simulink model "min_ord"  (R2025a)
settings: Solver=VariableStepAuto  StartTime=0.0  StopTime=50  RelTol=1e-3
values from neighbouring files (symbols this model uses):
  A_hat = Abb- Ke_obs*Aab    [Controls_proj.m]
  A_real = double(A_real)    [Controls_proj.m]
  B_hat = A_hat*Ke_obs + Aba - Ke_obs*Aaa    [Controls_proj.m]
  B_real = double(B_real)    [Controls_proj.m]
  C_hat = zeros(6, 4)    [Controls_proj.m]
  C_sens = [1 0 0 0 0 0 ; 0 0 1 0 0 0]    [Controls_proj.m]
  D_hat = zeros(6, 2)    [Controls_proj.m]
  F_hat = Bb -Ke_obs*Ba    [Controls_proj.m]
  K = lqr(A_real,B_real,Q,R_lqr)    [Controls_proj.m]
libraries: simulink x2
settings Model: Creator=retqrd  LastModifiedBy=retqrd

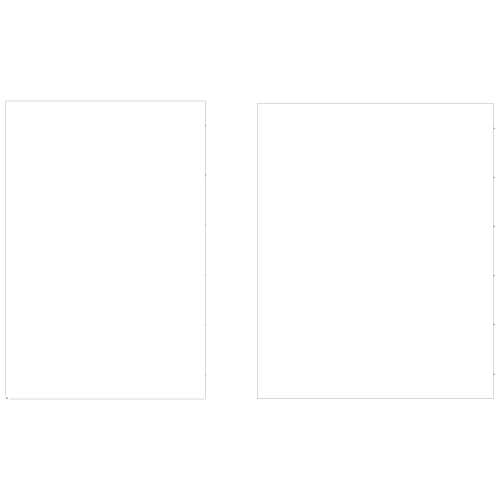
[thumbnail: Simulink's stored preview of the top-level diagram]
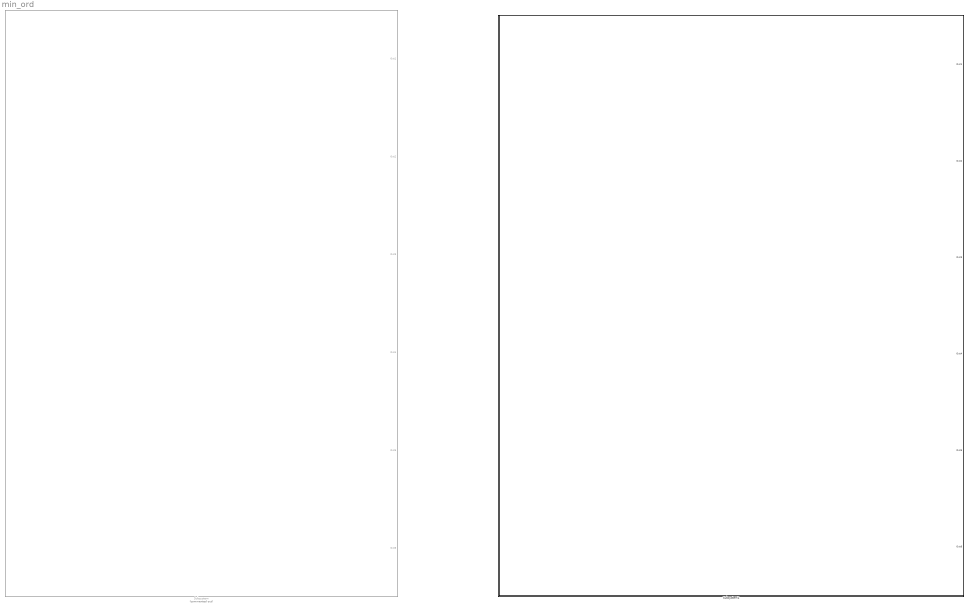
== system min_ord ==
  Subsystem : Subsystem  Commented=on
  Subsystem1 : Subsystem

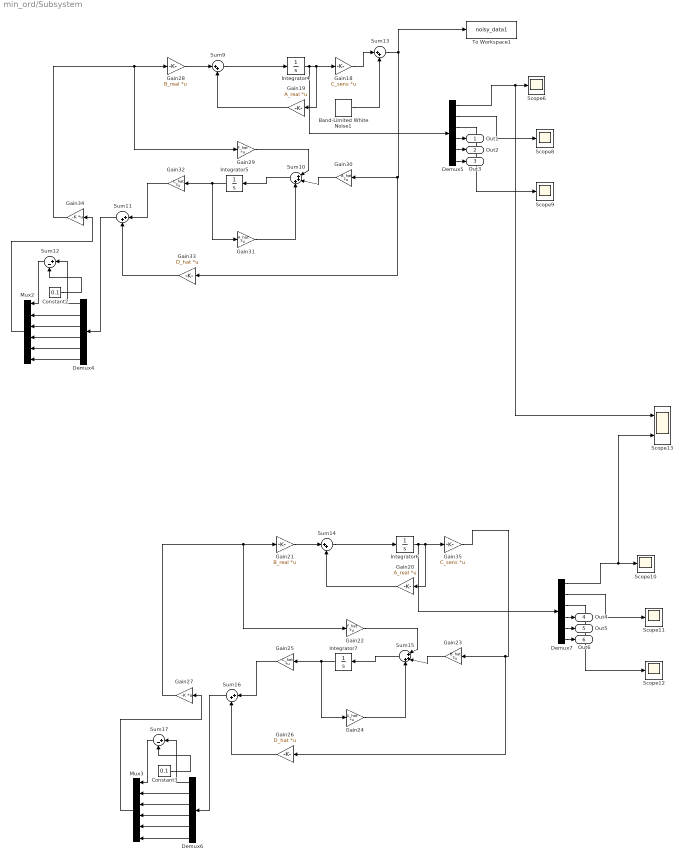
== system min_ord/Subsystem ==
  Band-Limited White Noise1 : simulink/Sources/Band-Limited White Noise  Cov=exp(-16)*[1 1]  Ts=0.001  seed=[23341 54321]
  Constant2 : Constant  Value=0.1
  Constant3 : Constant  Value=0.1
  Demux{4..7} (4 alike) : Demux  Outputs=6
  Gain18 : Gain  Gain=C_sens  Multiplication=Matrix(K*u)
  Gain19 : Gain  Gain=A_real  Multiplication=Matrix(K*u)
  Gain20 : Gain  Gain=A_real  Multiplication=Matrix(K*u)
  Gain21 : Gain  Gain=B_real  Multiplication=Matrix(K*u)
  Gain22 : Gain  Gain=F_hat  Multiplication=Matrix(K*u)
  Gain23 : Gain  Gain=B_hat  Multiplication=Matrix(K*u)
  Gain24 : Gain  Gain=A_hat  Multiplication=Matrix(K*u)
  Gain25 : Gain  Gain=C_hat  Multiplication=Matrix(K*u)
  Gain26 : Gain  Gain=D_hat  Multiplication=Matrix(K*u)
  Gain27 : Gain  Gain=-K  Multiplication=Matrix(K*u)
  Gain28 : Gain  Gain=B_real  Multiplication=Matrix(K*u)
  Gain29 : Gain  Gain=F_hat  Multiplication=Matrix(K*u)
  Gain30 : Gain  Gain=B_hat  Multiplication=Matrix(K*u)
  Gain31 : Gain  Gain=A_hat  Multiplication=Matrix(K*u)
  Gain32 : Gain  Gain=C_hat  Multiplication=Matrix(K*u)
  Gain33 : Gain  Gain=D_hat  Multiplication=Matrix(K*u)
  Gain34 : Gain  Gain=-K  Multiplication=Matrix(K*u)
  Gain35 : Gain  Gain=C_sens  Multiplication=Matrix(K*u)
  Integrator4 : Integrator  InitialCondition=[0;0;1*pi/180;0;0;0]
  Integrator5 : Integrator  InitialCondition=[0;0;0;0]
  Integrator6 : Integrator  InitialCondition=[0;0;1*pi/180;0;0;0]
  Integrator7 : Integrator  InitialCondition=[0;0;0;0]
  Mux2 : Mux  Inputs=6
  Mux3 : Mux  Inputs=6
  Scope{6,8..12} (6 alike) : Scope
      Scope10 settings: ActiveDisplayYMinimum=-1.4571930900555263  ActiveDisplayYMaximum=2.3047007119149248  DataLoggingVariableName=ScopeData6
      Scope11 settings: ActiveDisplayYMinimum=-38.619010005293767  ActiveDisplayYMaximum=75.841971632871335  DataLoggingVariableName=ScopeData8
      Scope12 settings: ActiveDisplayYMinimum=0.076583474303589763  ActiveDisplayYMaximum=0.25055600855879168  DataLoggingVariableName=ScopeData9
      Scope6 settings: ActiveDisplayYMinimum=-553.06616250271725  ActiveDisplayYMaximum=790.95216777342159  DataLoggingVariableName=ScopeData11
      Scope8 settings: ActiveDisplayYMinimum=-38.619010005293767  ActiveDisplayYMaximum=75.841971632871335  DataLoggingVariableName=ScopeData12
      Scope9 settings: ActiveDisplayYMinimum=0.076583474303589763  ActiveDisplayYMaximum=0.25055600855879168  DataLoggingVariableName=ScopeData13
  Scope13 : Scope  NumInputPorts=2
      settings: ActiveDisplayYMinimum=-66.910633005790316  ActiveDisplayYMaximum=43.530378748753677  DataLoggingVariableName=ScopeData10
  Sum10 : Sum  Inputs=|+++
  Sum{9,11,13..14,16} (5 alike) : Sum  Inputs=|++
  Sum12 : Sum  Inputs=|+-
  Sum15 : Sum  Inputs=|+++
  Sum17 : Sum  Inputs=|+-
  To Workspace1 : ToWorkspace  VariableName=noisy_data1  SampleTime=-1
  Out1 : Outport
  Out2 : Outport  Port=2
  Out3 : Outport  Port=3
  Out4 : Outport  Port=4
  Out5 : Outport  Port=5
  Out6 : Outport  Port=6
  wires:
  Band-Limited White Noise1/1 -> Sum13/2
  Gain22/1 -> Sum15/1
  Sum11/1 -> Demux4/1
  Gain29/1 -> Sum10/1
  Sum13/1 -> To Workspace1/1, Gain33/1, Gain30/1
  Sum10/1 -> Integrator5/1
  Demux6/2 -> Mux3/2
  Sum15/1 -> Integrator7/1
  Demux7/3 -> Scope12/1
  Demux5/4 -> Out1/1
  Integrator6/1 -> Demux7/1, Gain20/1, Gain35/1
  Gain32/1 -> Sum11/1
  Demux6/4 -> Mux3/4
  Demux6/1 -> Sum17/1
  Demux6/6 -> Mux3/6
  Mux3/1 -> Gain27/1
  Demux4/4 -> Mux2/4
  Sum14/1 -> Integrator6/1
  Demux7/6 -> Out6/1
  Demux5/2 -> Scope8/1
  Demux5/5 -> Out2/1
  Constant3/1 -> Sum17/2
  Integrator5/1 -> Gain31/1, Gain32/1
  Demux4/3 -> Mux2/3
  Sum16/1 -> Demux6/1
  Demux4/2 -> Mux2/2
  Gain31/1 -> Sum10/3
  Gain28/1 -> Sum9/1
  Mux2/1 -> Gain34/1
  Gain23/1 -> Sum15/2
  Demux6/3 -> Mux3/3
  Integrator7/1 -> Gain24/1, Gain25/1
  Demux5/1 -> Scope13/1, Scope6/1
  Sum17/1 -> Mux3/1
  Constant2/1 -> Sum12/2
  Demux7/5 -> Out5/1
  Demux7/4 -> Out4/1
  Demux6/5 -> Mux3/5
  Gain30/1 -> Sum10/2
  Demux4/1 -> Sum12/1
  Gain18/1 -> Sum13/1
  Gain35/1 -> Gain26/1, Gain23/1
  Demux4/5 -> Mux2/5
  Integrator4/1 -> Demux5/1, Gain19/1, Gain18/1
  Gain34/1 -> Gain29/1, Gain28/1
  Gain27/1 -> Gain22/1, Gain21/1
  Demux5/3 -> Scope9/1
  Gain33/1 -> Sum11/2
  Gain21/1 -> Sum14/1
  Demux7/1 -> Scope13/2, Scope10/1
  Gain19/1 -> Sum9/2
  Demux5/6 -> Out3/1
  Demux7/2 -> Scope11/1
  Gain25/1 -> Sum16/1
  Demux4/6 -> Mux2/6
  Sum9/1 -> Integrator4/1
  Gain24/1 -> Sum15/3
  Gain26/1 -> Sum16/2
  Sum12/1 -> Mux2/1
  Gain20/1 -> Sum14/2

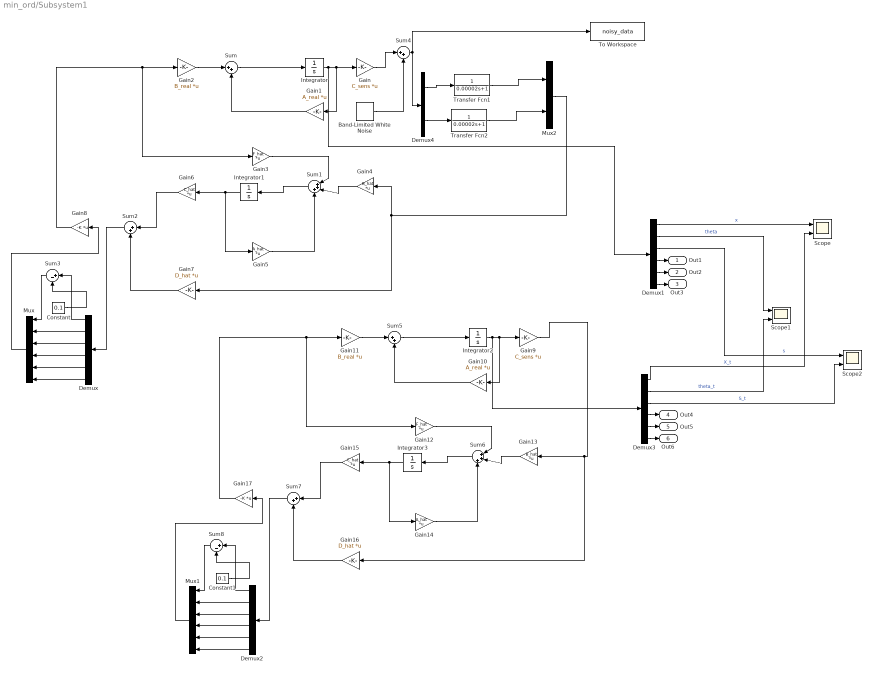
== system min_ord/Subsystem1 ==
  Band-Limited White Noise : simulink/Sources/Band-Limited White Noise  Cov=exp(-16)*[1 1]  Ts=0.001  seed=[23341 54321]
  Constant : Constant  Value=0.1
  Constant1 : Constant  Value=0.1
  Demux{,1..3} (4 alike) : Demux  Outputs=6
  Demux4 : Demux  Outputs=2
  Gain : Gain  Gain=C_sens  Multiplication=Matrix(K*u)
  Gain1 : Gain  Gain=A_real  Multiplication=Matrix(K*u)
  Gain10 : Gain  Gain=A_real  Multiplication=Matrix(K*u)
  Gain11 : Gain  Gain=B_real  Multiplication=Matrix(K*u)
  Gain12 : Gain  Gain=F_hat  Multiplication=Matrix(K*u)
  Gain13 : Gain  Gain=B_hat  Multiplication=Matrix(K*u)
  Gain14 : Gain  Gain=A_hat  Multiplication=Matrix(K*u)
  Gain15 : Gain  Gain=C_hat  Multiplication=Matrix(K*u)
  Gain16 : Gain  Gain=D_hat  Multiplication=Matrix(K*u)
  Gain17 : Gain  Gain=-K  Multiplication=Matrix(K*u)
  Gain2 : Gain  Gain=B_real  Multiplication=Matrix(K*u)
  Gain3 : Gain  Gain=F_hat  Multiplication=Matrix(K*u)
  Gain4 : Gain  Gain=B_hat  Multiplication=Matrix(K*u)
  Gain5 : Gain  Gain=A_hat  Multiplication=Matrix(K*u)
  Gain6 : Gain  Gain=C_hat  Multiplication=Matrix(K*u)
  Gain7 : Gain  Gain=D_hat  Multiplication=Matrix(K*u)
  Gain8 : Gain  Gain=-K  Multiplication=Matrix(K*u)
  Gain9 : Gain  Gain=C_sens  Multiplication=Matrix(K*u)
  Integrator : Integrator  InitialCondition=[0;0;4*pi/180;0;0;0]
  Integrator1 : Integrator  InitialCondition=[0;0;0;0]
  Integrator2 : Integrator  InitialCondition=[0;0;4*pi/180;0;0;0]
  Integrator3 : Integrator  InitialCondition=[0;0;0;0]
  Mux : Mux  Inputs=6
  Mux1 : Mux  Inputs=6
  Mux2 : Mux  Inputs=2
  Scope : Scope  NumInputPorts=2
  Scope1 : Scope  NumInputPorts=2
  Scope2 : Scope  NumInputPorts=2
      settings: ActiveDisplayYMinimum=-2.5105740742429736  ActiveDisplayYMaximum=1.9646271868821386  DataLoggingVariableName=ScopeData2
  Sum{,2,4..5,7} (5 alike) : Sum  Inputs=|++
  Sum1 : Sum  Inputs=|+++
  Sum3 : Sum  Inputs=|+-
  Sum6 : Sum  Inputs=|+++
  Sum8 : Sum  Inputs=|+-
  To Workspace : ToWorkspace  VariableName=noisy_data  SampleTime=-1
  Transfer Fcn1 : TransferFcn  Denominator=[0.00002 1]
  Transfer Fcn2 : TransferFcn  Denominator=[0.00002 1]
  Out1 : Outport
  Out2 : Outport  Port=2
  Out3 : Outport  Port=3
  Out4 : Outport  Port=4
  Out5 : Outport  Port=5
  Out6 : Outport  Port=6
  wires:
  Demux/4 -> Mux/4
  Sum5/1 -> Integrator2/1
  Gain12/1 -> Sum6/1
  Demux/2 -> Mux/2
  Sum8/1 -> Mux1/1
  Gain13/1 -> Sum6/2
  Gain7/1 -> Sum2/2
  Gain14/1 -> Sum6/3
  Demux2/5 -> Mux1/5
  Gain15/1 -> Sum7/1
  Integrator/1 -> Demux1/1, Gain1/1, Gain/1
  Constant1/1 -> Sum8/2
  Sum6/1 -> Integrator3/1
  Constant/1 -> Sum3/2
  Gain2/1 -> Sum/1
  Gain17/1 -> Gain12/1, Gain11/1
  Demux3/5 -> Out5/1
  Demux2/1 -> Sum8/1
  Demux1/6 -> Out3/1
  Demux2/6 -> Mux1/6
  Gain3/1 -> Sum1/1
  Mux2/1 -> Gain4/1, Gain7/1
  Gain10/1 -> Sum5/2
  Gain9/1 -> Gain16/1, Gain13/1
  Sum4/1 -> Demux4/1, To Workspace/1
  Sum7/1 -> Demux2/1
  Mux/1 -> Gain8/1
  Demux2/4 -> Mux1/4
  Integrator1/1 -> Gain5/1, Gain6/1
  Sum2/1 -> Demux/1
  Mux1/1 -> Gain17/1
  Sum/1 -> Integrator/1
  Gain16/1 -> Sum7/2
  Demux/5 -> Mux/5
  Demux/6 -> Mux/6
  Demux/1 -> Sum3/1
  Demux3/4 -> Out4/1
  Gain1/1 -> Sum/2
  Demux2/3 -> Mux1/3
  Gain11/1 -> Sum5/1
  Integrator3/1 -> Gain14/1, Gain15/1
  Sum3/1 -> Mux/1
  Integrator2/1 -> Demux3/1, Gain10/1, Gain9/1
  Transfer Fcn2/1 -> Mux2/2
  Demux1/5 -> Out2/1
  Gain6/1 -> Sum2/1
  Gain4/1 -> Sum1/2
  Demux/3 -> Mux/3
  Transfer Fcn1/1 -> Mux2/1
  Demux3/6 -> Out6/1
  Demux1/4 -> Out1/1
  Gain8/1 -> Gain3/1, Gain2/1
  Band-Limited White Noise/1 -> Sum4/2
  Demux4/2 -> Transfer Fcn2/1
  Gain/1 -> Sum4/1
  Sum1/1 -> Integrator1/1
  Gain5/1 -> Sum1/3
  Demux4/1 -> Transfer Fcn1/1
  Demux2/2 -> Mux1/2
  Demux1/1 -> Scope/1  "x"
  Demux3/1 -> Scope/2  "X_t"
  Demux1/2 -> Scope1/1  "theta"
  Demux3/2 -> Scope1/2  "theta_t"
  Demux1/3 -> Scope2/1  "s"
  Demux3/3 -> Scope2/2  "S_t"
